simulink model "CovPredTestHarness"  (Simulink 7.9)
settings: Solver=FixedStepDiscrete  StartTime=0.0  StopTime=1  FixedStep=1  RelTol=1e-3
values from neighbouring files (symbols this model uses):
  correctedDelAng = double(correctedDelAng)    [SaveCovPredTestData.m]
  correctedDelVel = double(correctedDelVel)    [SaveCovPredTestData.m]
  dt = median(diff(StateDataOut(:,1)))    [PlotCcodeOutput.m]    (also in ReadCovPredTestHarnessFiles.m = fscanf (fid, '; SaveCovPredTestData.m = double(dt))
  onGround = boolean(fscanf (fid, '    [ReadCovPredTestHarnessFiles.m]    (also in SaveCovPredTestData.m = double(onGround))
  Pin = zeros(24,24)    [ReadCovPredTestHarnessFiles.m]    (also in SaveCovPredTestData.m = double(Pin))
  states = double(states)    [SaveCovPredTestData.m]
  useAirspeed = boolean(fscanf (fid, '    [ReadCovPredTestHarnessFiles.m]    (also in SaveCovPredTestData.m = double(useAirspeed))
  useCompass = boolean(fscanf (fid, '    [ReadCovPredTestHarnessFiles.m]    (also in SaveCovPredTestData.m = double(useCompass))
(part 1 of 2)
settings Model: Creator=user  LastModifiedBy=user

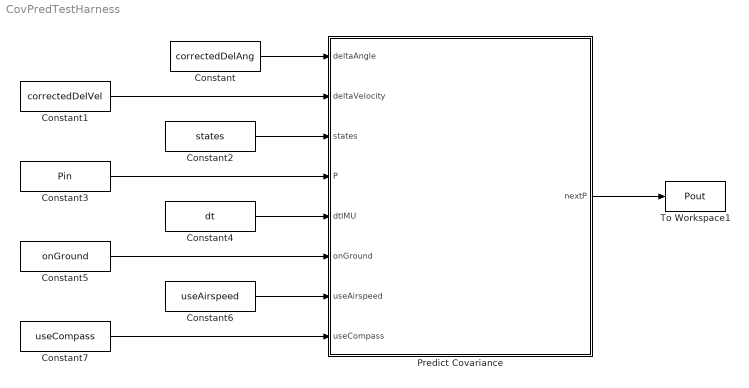
== system CovPredTestHarness ==
  Constant : Constant  Value=correctedDelAng  OutDataTypeStr=double
  Constant1 : Constant  Value=correctedDelVel  OutDataTypeStr=double
  Constant2 : Constant  Value=states  OutDataTypeStr=double
  Constant3 : Constant  Value=Pin  OutDataTypeStr=double
  Constant4 : Constant  Value=dt  OutDataTypeStr=double
  Constant5 : Constant  Value=onGround  OutDataTypeStr=boolean
  Constant6 : Constant  Value=useAirspeed  OutDataTypeStr=boolean
  Constant7 : Constant  Value=useCompass  OutDataTypeStr=boolean
  Predict Covariance : MATLAB Function  TreatAsAtomicUnit=on
  To Workspace1 : ToWorkspace  VariableName=Pout  SampleTime=-1
      settings: MaxDataPoints=1
  wires:
  Constant/1 -> Predict Covariance/1(deltaAngle)
  Constant1/1 -> Predict Covariance/2(deltaVelocity)
  Constant2/1 -> Predict Covariance/3(states)
  Constant3/1 -> Predict Covariance/4(P)
  Constant4/1 -> Predict Covariance/5(dtIMU)
  Constant5/1 -> Predict Covariance/6(onGround)
  Constant6/1 -> Predict Covariance/7(useAirspeed)
  Constant7/1 -> Predict Covariance/8(useCompass)
  Predict Covariance/1(nextP) -> To Workspace1/1
